simulink model "rosmca3"  (Simulink 8.5)
settings: Solver=ode45  StartTime=0.0  StopTime=2000  RelTol=1e-6
libraries: simulink x3
settings Model: Creator=dercole  LastModifiedBy=Alessandra  ExtModeTrigMode=oneshot  ExtModeArmWhenConnect=off  ExtModeAutoUpdateStatusClock=off
settings DataIOCC: LimitDataPoints=off
settings OptimizationCC: BooleanDataType=off  ExpressionDepthLimit=128
settings DebuggingCC: SaveWithParameterizedLinksMsg=none  SignalResolutionControl=TryResolveAllWithWarning  MultiTaskDSMMsg=warning  MultiTaskCondExecSysMsg=none  FcnCallInpInsideContextMsg=EnableAllAsError  StateNameClashWarn=none
settings HardwareCC: TargetUnknown=on

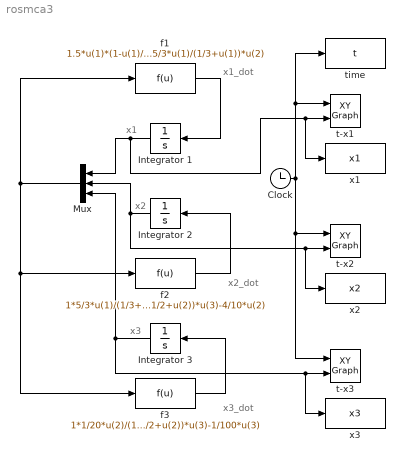
== system rosmca3 ==
  note: x1_dot
  note: x3_dot
  note: x3
  note: x1
  note: x2_dot
  note: x2
  Clock : Clock
  Integrator 1 : Integrator  InitialCondition=1
  "Integrator 2 " : Integrator  InitialCondition=1
  Integrator 3 : Integrator  InitialCondition=10
  Mux : Mux  Inputs=3
  f1 : Fcn  Expr=1.5*u(1)*(1-u(1)/1)-5/3*u(1)/(1/3+u(1))*u(2)
  f2 : Fcn  Expr=1*5/3*u(1)/(1/3+u(1))*u(2)-1/20*u(2)/(1/2+u(2))*u(3)-4/10*u(2)
  f3 : Fcn  Expr=1*1/20*u(2)/(1/2+u(2))*u(3)-1/100*u(3)
  t-x1 : simulink/Sinks/XY Graph  xmin=0  xmax=2000  ymin=0  ymax=2  st=-1
  t-x2 : simulink/Sinks/XY Graph  xmin=0  xmax=2000  ymin=0  ymax=2  st=-1
  t-x3 : simulink/Sinks/XY Graph  xmin=0  xmax=2000  ymin=0  ymax=15  st=-1
  time : ToWorkspace  VariableName=t  SampleTime=-1
  x1 : ToWorkspace  VariableName=x1  SampleTime=-1
  x2 : ToWorkspace  VariableName=x2  SampleTime=-1
  x3 : ToWorkspace  VariableName=x3  SampleTime=-1
  wires:
  f1/1 -> Integrator 1/1
  f3/1 -> Integrator 3/1
  Mux/1 -> f1/1, f3/1, f2/1
  Integrator 1/1 -> Mux/1, t-x1/2, x1/1
  Clock/1 -> t-x2/1, t-x3/1, t-x1/1, time/1
  Integrator 3/1 -> Mux/3, t-x3/2, x3/1
  f2/1 -> "Integrator 2 "/1
  "Integrator 2 "/1 -> Mux/2, t-x2/2, x2/1
